simulink model "suspensionPE"  (R2015a)
settings: Solver=ode23t  StartTime=0.0  StopTime=60  RelTol=1e-3  AbsTol=1e-3
PreLoadFcn:
  | load carParams
  | k1 = 100000;
  | k2 = 100000;
  | b1 = 1000;
  | b2 = 1000;
libraries: fl_lib x9, nesl_utility x3
settings Model: Creator=scastro  LastModifiedBy=chahn
settings DataIOCC: LimitDataPoints=off  OutputTimes=0:0.01:60
settings SimscapeCC: SimscapeLogDataHistory=10000

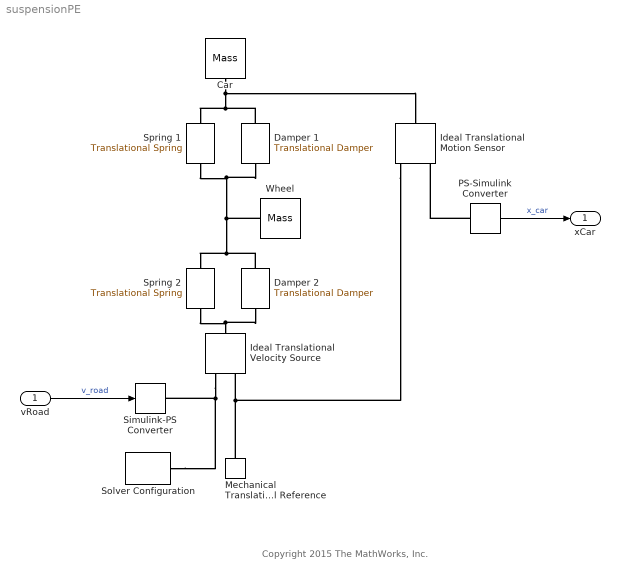
== system suspensionPE ==
  note: Copyright 2015 The MathWorks, Inc.
  vRoad : Inport
  Car : fl_lib/Mechanical/Translational Elements/Mass  mass=mCar kg  v_specify=off  v_priority=High  v=0 m/s  f_specify=off  f_priority=High  f=0 N
  Damper 1 : fl_lib/Mechanical/Translational Elements/Translational Damper  D=b1 N/(m/s)  v_specify=off  v_priority=High  v=0 m/s  f_specify=off  f_priority=High  f=0 N
  Damper 2 : fl_lib/Mechanical/Translational Elements/Translational Damper  D=b2 N/(m/s)  v_specify=off  v_priority=High  v=0 m/s  f_specify=off  f_priority=High  f=0 N
  Ideal Translational Motion Sensor : fl_lib/Mechanical/Mechanical Sensors/Ideal Translational Motion Sensor  offset=0 m
  Ideal Translational Velocity Source : fl_lib/Mechanical/Mechanical Sources/Ideal Translational Velocity Source
  Mechanical Translational Reference : fl_lib/Mechanical/Translational Elements/Mechanical Translational Reference
  PS-Simulink Converter : nesl_utility/PS-Simulink Converter  PhysicalDomain=network_engine_domain  SubClassName=ps_output  LeftPortType=input  RightPortType=output  PseudoPeriodic=off  Frequencies=[]  Unit=cm  AffineConversion=off
  Simulink-PS Converter : nesl_utility/Simulink-PS Converter  PhysicalDomain=network_engine_domain  SubClassName=ps_input  LeftPortType=input  RightPortType=output  PseudoPeriodic=off  Frequencies=[]  NoiseDistribution=none  NoiseParameters=[]  Unit=cm/s  AffineConversion=off  InputFiltering=off  SimscapeFilterOrder=1  InputFilterTimeConstant=0.001  UdotUserProvided=1
  Solver Configuration : nesl_utility/Solver Configuration  PhysicalDomain=network_engine_domain  SubClassName=solver  LeftPortType=input  RightPortType=generic  Accelerate=off  Tones=[]  Harmonics=[]  SimulateNoise=off  Profile=off  UseLocalSampling=off  EnableSwitchedLinearOptims=on  FrequencyDomain=off  UseCCode=off  RelTol=0.001  AbsTol=1e-06  MinStep=1e-09  ToWorkspace=off  RevertToSquareIcSolve=off  NumHomotopyIterations=100  DoDC=off  ResidualTolerance=1e-09  UseLocalSolver=off  LocalSolverChoice=NE_BACKWARD_EULER_ADVANCER  LocalSolverSampleTime=0.001  DoFixedCost=off  MaxNonlinIter=3  MaxModeIter=2  LinearAlgebra=Sparse  DelaysMemoryBudget=1024  AutomaticFiltering=on  FilteringTimeConstant=0.001
  Spring 1 : fl_lib/Mechanical/Translational Elements/Translational Spring  spr_rate=k1 N/m  v_specify=off  v_priority=High  v=0 m/s  f_specify=off  f_priority=High  f=0 N  x_specify=off  x_priority=High  x=0 m
  Spring 2 : fl_lib/Mechanical/Translational Elements/Translational Spring  spr_rate=k2 N/m  v_specify=off  v_priority=High  v=0 m/s  f_specify=off  f_priority=High  f=0 N  x_specify=off  x_priority=High  x=0 m
  Wheel : fl_lib/Mechanical/Translational Elements/Mass  mass=mWheel kg  v_specify=off  v_priority=High  v=0 m/s  f_specify=off  f_priority=High  f=0 N
  xCar : Outport
  wires:
  vRoad/1 -> Simulink-PS Converter/1  "v_road"
  PS-Simulink Converter/1 -> xCar/1  "x_car"
  connections:
  Ideal Translational Velocity Source/RConn1 -- Solver Configuration/RConn1 -- Simulink-PS Converter/RConn1
  Mechanical Translational Reference/LConn1 -- Ideal Translational Motion Sensor/RConn1 -- Ideal Translational Velocity Source/RConn2
  Spring 2/RConn1 -- Damper 2/RConn1 -- Ideal Translational Velocity Source/LConn1
  Damper 1/RConn1 -- Spring 1/RConn1 -- Spring 2/LConn1 -- Damper 2/LConn1 -- Wheel/LConn1
  Spring 1/LConn1 -- Ideal Translational Motion Sensor/LConn1 -- Car/LConn1 -- Damper 1/LConn1
  PS-Simulink Converter/LConn1 -- Ideal Translational Motion Sensor/RConn3
